simulink model "complete_controller_masterslave"  (R2016a)
settings: Solver=FixedStepAuto  StartTime=0.0  StopTime=50  FixedStep=0.1  RelTol=1e-3
settings Model: ExtModeTrigDuration=5  Creator=aless  LastModifiedBy=aless
settings OptimizationCC: DefaultParameterBehavior=Inlined  OptimizeModelRefInitCode=on  LifeSpan=1
settings HardwareCC: ProdBitPerPointer=32  ProdLargestAtomicInteger=Long  ProdLargestAtomicFloat=Double  ProdWordSize=32  ProdHWDeviceType=ARM Compatible->ARM Cortex
settings RTWCC: SystemTargetFile=ert.tlc  GenCodeOnly=on  TemplateMakefile=ert_default_tmf  GenerateReport=on  IncludeHyperlinkInReport=on  LaunchReport=on  GenerateTraceInfo=on  GenerateTraceReport=on  GenerateTraceReportSl=on  GenerateTraceReportSf=on  GenerateTraceReportEml=on
settings CodeAppCC: ForceParamTrailComments=on  OperatorAnnotations=on  SimulinkDataObjDesc=on  SFDataObjDesc=on  MATLABFcnDesc=on  InsertBlockDesc=on  MATLABSourceComments=on
settings ERTTargetCC: GenerateSampleERTMain=on  MultiInstanceERTCode=on  CodeInterfacePackaging=Reusable function  InlinedParameterPlacement=NonHierarchical  RootIOFormat=Structure reference  ERTCustomFileTemplate=example_file_process.tlc  ERTFilePackagingFormat=Compact

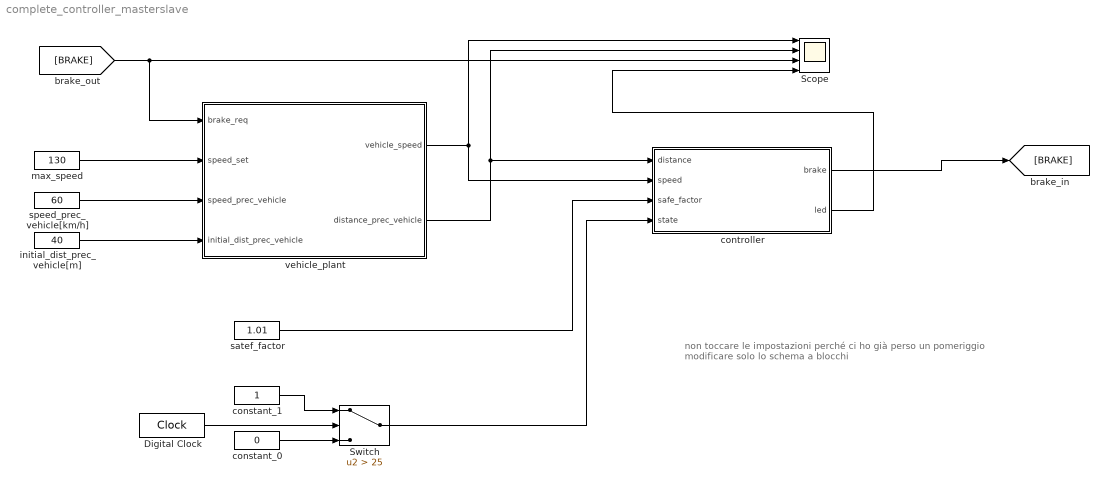
== system complete_controller_masterslave ==
  note: non toccare le impostazioni perché ci ho già perso un pomeriggio
      | modificare solo lo schema a blocchi
  Digital Clock : DigitalClock  SampleTime=0.1
  Scope : Scope  NumInputPorts=4
  Switch : Switch  Criteria=u2 > Threshold  Threshold=25
  constant_0 : Constant  Value=0
  constant_1 : Constant
  controller : Subsystem
  initial_dist_prec_vehicle[m] : Constant  Value=40
  max_speed : Constant  Value=130
  satef_factor : Constant  Value=1.01
  speed_prec_vehicle[km/h] : Constant  Value=60
  vehicle_plant : Subsystem
  wires:
  vehicle_plant/1(vehicle_speed) -> controller/2(speed), Scope/1
  vehicle_plant/2(distance_prec_vehicle) -> Scope/2, controller/1(distance)
  max_speed/1 -> vehicle_plant/2(speed_set)
  initial_dist_prec_vehicle[m]/1 -> vehicle_plant/4(initial_dist_prec_vehicle)
  speed_prec_vehicle[km/h]/1 -> vehicle_plant/3(speed_prec_vehicle)
  [BRAKE] -> vehicle_plant/1(brake_req), Scope/3
  controller/1(brake) -> [BRAKE]
  controller/2(led) -> Scope/4
  satef_factor/1 -> controller/3(safe_factor)
  Switch/1 -> controller/4(state)
  Digital Clock/1 -> Switch/2
  constant_0/1 -> Switch/3
  constant_1/1 -> Switch/1

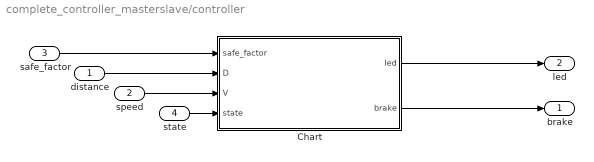
== system complete_controller_masterslave/controller ==
  distance : Inport
  speed : Inport  Port=2
  safe_factor : Inport  Port=3
  state : Inport  Port=4
  Chart : Stateflow chart  TreatAsAtomicUnit=on
  brake : Outport
  led : Outport  Port=2
  wires:
  distance/1 -> Chart/2(D)
  speed/1 -> Chart/3(V)
  safe_factor/1 -> Chart/1(safe_factor)
  Chart/1(led) -> led/1
  Chart/2(brake) -> brake/1
  state/1 -> Chart/4(state)

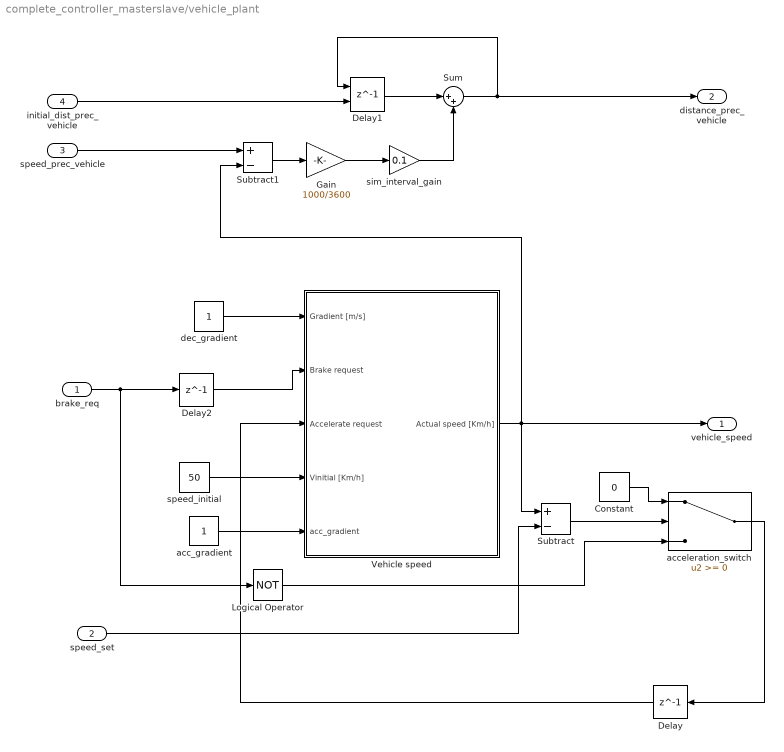
== system complete_controller_masterslave/vehicle_plant ==
  brake_req : Inport
  speed_set : Inport  Port=2
  speed_prec_vehicle : Inport  Port=3
  initial_dist_prec_vehicle : Inport  Port=4
  Constant : Constant  Value=0
  Delay : Delay  DelayLength=1  InitialCondition=0
  Delay1 : Delay  DelayLength=1  InitialConditionSource=Input port  InitialCondition=0
      settings: InputPortMap=u0,p4
  Delay2 : Delay  DelayLength=1  InitialCondition=0
  Gain : Gain  Gain=1000/3600
  Logical Operator : Logic  Operator=NOT  AllPortsSameDT=off  OutDataTypeStr=boolean
  Subtract : Sum  Inputs=+-
  Subtract1 : Sum  Inputs=+-
  Sum : Sum  Inputs=|++
  Vehicle speed : Subsystem
  acc_gradient : Constant
  acceleration_switch : Switch  RndMeth=Nearest
  dec_gradient : Constant
  sim_interval_gain : Gain  Gain=0.1
  speed_initial : Constant  Value=50
  vehicle_speed : Outport
  distance_prec_vehicle : Outport  Port=2
  wires:
  dec_gradient/1 -> Vehicle speed/1(Gradient [m/s])
  speed_initial/1 -> Vehicle speed/4(Vinitial [Km/h])
  Vehicle speed/1(Actual speed [Km/h]) -> vehicle_speed/1, Subtract1/2, Subtract/1
  Constant/1 -> acceleration_switch/1
  brake_req/1 -> Logical Operator/1, Delay2/1
  acceleration_switch/1 -> Delay/1
  Subtract/1 -> acceleration_switch/2
  speed_set/1 -> Subtract/2
  speed_prec_vehicle/1 -> Subtract1/1
  Subtract1/1 -> Gain/1
  Sum/1 -> distance_prec_vehicle/1, Delay1/1
  initial_dist_prec_vehicle/1 -> Delay1/2
  Delay1/1 -> Sum/1
  Gain/1 -> sim_interval_gain/1
  sim_interval_gain/1 -> Sum/2
  Delay2/1 -> Vehicle speed/2(Brake request)
  Logical Operator/1 -> acceleration_switch/3
  acc_gradient/1 -> Vehicle speed/5(acc_gradient)
  Delay/1 -> Vehicle speed/3(Accelerate request)

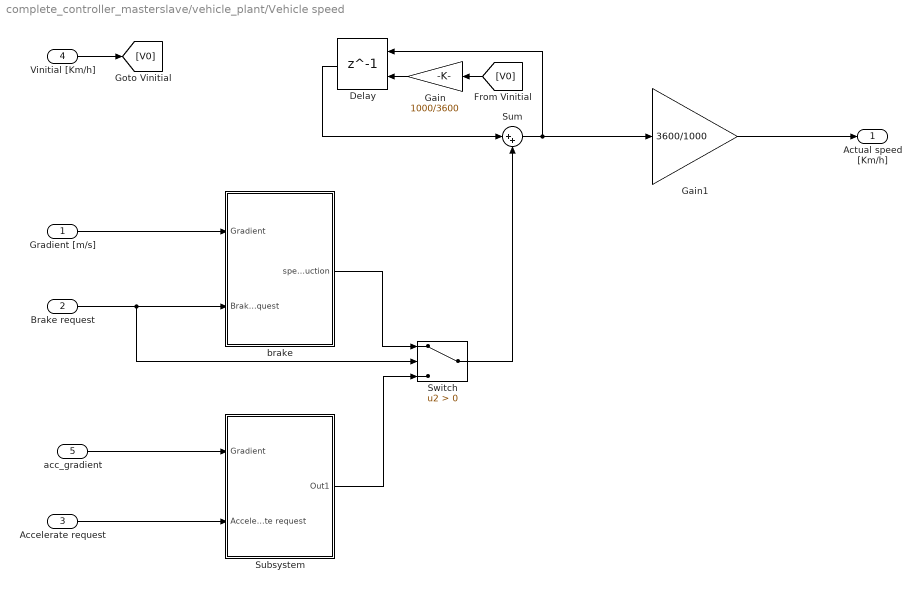
== system complete_controller_masterslave/vehicle_plant/Vehicle speed ==
  Gradient [m/s] : Inport
  Brake request : Inport  Port=2
  Accelerate request : Inport  Port=3
  Vinitial [Km/h] : Inport  Port=4
  acc_gradient : Inport  Port=5
  Delay : Delay  DelayLength=1  InitialConditionSource=Input port  InitialCondition=0
      settings: InputPortMap=u0,p4
  Gain : Gain  Gain=1000/3600
  Gain1 : Gain  Gain=3600/1000
  Subsystem : Subsystem
  Sum : Sum  Inputs=|++
  Switch : Switch  Criteria=u2 > Threshold
  brake : Subsystem
  Actual speed [Km/h] : Outport
  wires:
  Brake request/1 -> Switch/2, brake/2(Brake request)
  Gradient [m/s]/1 -> brake/1(Gradient)
  Gain/1 -> Delay/2
  Subsystem/1(Out1) -> Switch/3
  Gain1/1 -> Actual speed [Km/h]/1
  Switch/1 -> Sum/2
  Accelerate request/1 -> Subsystem/2(Acceleate request)
  brake/1(speed_reduction) -> Switch/1
  Sum/1 -> Gain1/1, Delay/1
  [V0] -> Gain/1
  Delay/1 -> Sum/1
  Vinitial [Km/h]/1 -> [V0]
  acc_gradient/1 -> Subsystem/1(Gradient)

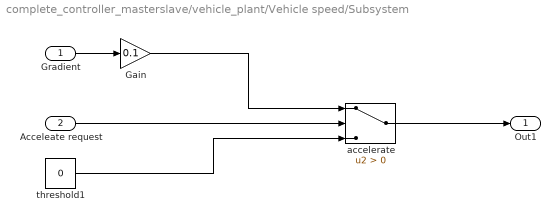
== system complete_controller_masterslave/vehicle_plant/Vehicle speed/Subsystem ==
  Gradient : Inport
  Acceleate request : Inport  Port=2
  Gain : Gain  Gain=0.1
  accelerate : Switch  Criteria=u2 > Threshold
  threshold1 : Constant  Value=0
  Out1 : Outport
  wires:
  accelerate/1 -> Out1/1
  Acceleate request/1 -> accelerate/2
  Gradient/1 -> Gain/1
  threshold1/1 -> accelerate/3
  Gain/1 -> accelerate/1

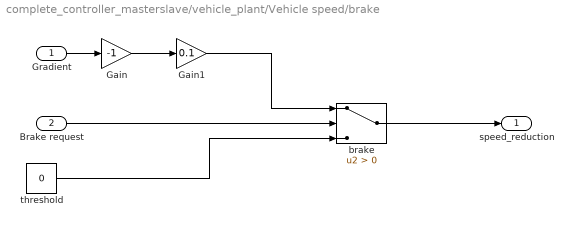
== system complete_controller_masterslave/vehicle_plant/Vehicle speed/brake ==
  Gradient : Inport
  Brake request : Inport  Port=2
  Gain : Gain  Gain=-1
  Gain1 : Gain  Gain=0.1
  brake : Switch  Criteria=u2 > Threshold
  threshold : Constant  Value=0
  speed_reduction : Outport
  wires:
  Gain/1 -> Gain1/1
  Gradient/1 -> Gain/1
  Gain1/1 -> brake/1
  Brake request/1 -> brake/2
  threshold/1 -> brake/3
  brake/1 -> speed_reduction/1

== stateflow chart complete_controller_masterslave/controller/Chart ==
  state INIT_STATE
    en: brake = uint8(0),
    led = uint8(0);
  state UNSAFE_DISTANCE
    en: brake = uint8(1);
    state LED_ON
      en: led = uint8(1);
    state LED_OFF
      en: led = uint8(0);
    (default) -> LED_ON
    LED_OFF -> LED_ON : after(1/(1+V^2/100-D), msec)
    LED_ON -> LED_OFF : after(1/(1+V^2/100-D), msec)
  state SAFE_DISTANCE
    en: brake = uint8(0),
    led = uint8(0);
  state MALFUNCTION
    en: brake = uint8(0),
    led = uint8(0);
  (default) -> INIT_STATE
  INIT_STATE -> UNSAFE_DISTANCE [order 2] : [(D <= (V^2)/100) && state ~= 1]
  INIT_STATE -> SAFE_DISTANCE [order 1] : [(D > (V^2)/100) && state ~= 1]
  INIT_STATE -> MALFUNCTION [order 3] : [state == 1]
  SAFE_DISTANCE -> UNSAFE_DISTANCE [order 1] : [(D <= (V^2)/100) && state ~= 1]
  UNSAFE_DISTANCE -> SAFE_DISTANCE [order 1] : [(D > (V^2)/100 * safe_factor) && state ~= 1]
  SAFE_DISTANCE -> MALFUNCTION [order 2] : [state == 1]
  UNSAFE_DISTANCE -> MALFUNCTION [order 2] : [state == 1]
  data: led output; safe_factor input; brake output; D input; V input; state input
